simulink model "WaterRocket_uebung"  (Simulink 8.9)
settings: Solver=ode45  StartTime=0.0  StopTime=20  FixedStep=0.000001  RelTol=1e-3  EnableMultiTasking=on
values from neighbouring files (symbols this model uses):
  A = [0 1 0;0 0 1; 0 0 0]    [KalmanBSP.m]    (also in ReadARISData.m = [0 1 0 0 0; 0 0 1 0 0; 0 0 0 0 0;0 0 0 0 0;-0.00649 0 0 0 0]; SEFromData.m = [0 1 0 0 0; SEFromDataWithGPS.m; SEFromDataWithPressure.m = [0 1 0 0 0 0;0 0 1 0 0 0; 0 0 0 0 0 0;0 PressLookUp(1,1) 0 0)
  airdensity = 1.204    [Wasserrakete_uebung.m]
  cw = 0.4    [Wasserrakete_uebung.m]
  F = 0.01^2*pi    (= 0.000314159265359)    [Wasserrakete_uebung.m]
  g = 9.807    [CalcPressure.m]    (also in KalmanBSP.m = 9.81; Wasserrakete_uebung.m = 9.81)
  h0 = 0.3    [Wasserrakete_uebung.m]
  kappa = 1.35    [Wasserrakete_uebung.m]
  ml = 0.113    [Wasserrakete_uebung.m]
  mw0 = v_opt*Vl*rho    (= 0)    [Wasserrakete_uebung.m]
  p0 = 4e5    (= 400000)    [Wasserrakete_uebung.m]
  pa = 0.97e5    (= 97000)    [Wasserrakete_uebung.m]
  rho = 1000    [Wasserrakete_uebung.m]
  V0 = Vl-mw0/rho    (= 0.00158)    [Wasserrakete_uebung.m]
  v0 = 0.0    (= 0)    [Wasserrakete_uebung.m]
  Vl = 1.58e-3    (= 0.00158)    [Wasserrakete_uebung.m]
settings Model: Creator=Benedikt Imbach  LastModifiedBy=Beda Föhn
settings OptimizationCC: InitFltsAndDblsToZero=on
settings DebuggingCC: SaveWithParameterizedLinksMsg=none  SolverPrmCheckMsg=warning
settings HardwareCC: TargetHWDeviceType=32-bit Generic
settings GRTTargetCC: TargetFcnLib=ansi_tfl_tmw.mat  GeneratePreprocessorConditionals=Use local settings

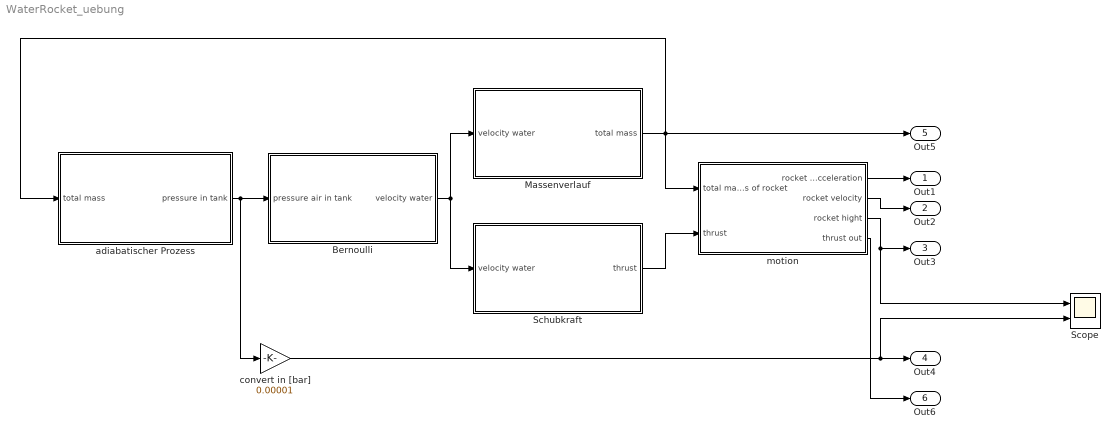
== system WaterRocket_uebung ==
  Bernoulli : Subsystem
  Massenverlauf : Subsystem
  Schubkraft : Subsystem
  Scope : Scope  NumInputPorts=2
  adiabatischer Prozess : Subsystem
  convert in [bar] : Gain  Gain=0.00001
  motion : Subsystem
  Out1 : Outport
  Out2 : Outport  Port=2
  Out3 : Outport  Port=3
  Out4 : Outport  Port=4
  Out5 : Outport  Port=5
  Out6 : Outport  Port=6
  wires:
  adiabatischer Prozess/1(pressure in tank) -> Bernoulli/1(pressure air in tank), convert in [bar]/1
  Bernoulli/1(velocity water) -> Massenverlauf/1(velocity water), Schubkraft/1(velocity water)
  Massenverlauf/1(total mass) -> motion/1(total mass of rocket), adiabatischer Prozess/1(total mass), Out5/1
  Schubkraft/1(thrust) -> motion/2(thrust)
  motion/1(rocket acceleration) -> Out1/1
  motion/2(rocket velocity) -> Out2/1
  motion/3(rocket hight) -> Scope/1, Out3/1
  motion/4(thrust out) -> Out6/1
  convert in [bar]/1 -> Scope/2, Out4/1

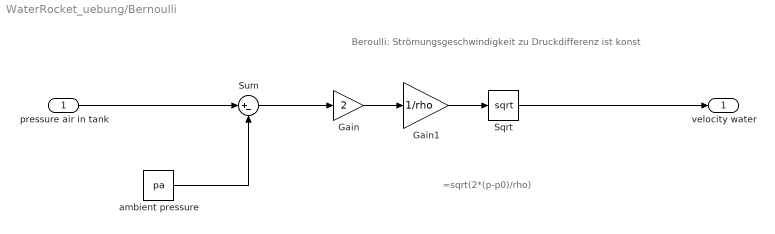
== system WaterRocket_uebung/Bernoulli ==
  note: =sqrt(2*(p-p0)/rho)
  note: Beroulli: Strömungsgeschwindigkeit zu Druckdifferenz ist konst
  pressure air in tank : Inport
  Gain : Gain  Gain=2
  Gain1 : Gain  Gain=1/rho
  Sqrt : Sqrt  SaturateOnIntegerOverflow=on
  Sum : Sum  Inputs=|+-
  ambient pressure : Constant  Value=pa
  velocity water : Outport
  wires:
  pressure air in tank/1 -> Sum/1
  ambient pressure/1 -> Sum/2
  Sum/1 -> Gain/1
  Gain/1 -> Gain1/1
  Gain1/1 -> Sqrt/1
  Sqrt/1 -> velocity water/1

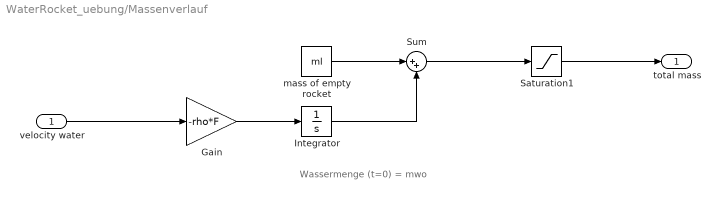
== system WaterRocket_uebung/Massenverlauf ==
  note: Wassermenge (t=0) = mwo
  velocity water : Inport
  Gain : Gain  Gain=-rho*F
  Integrator : Integrator  InitialCondition=mw0
  Saturation1 : Saturate  UpperLimit=ml+mw0  LowerLimit=ml
  Sum : Sum  Inputs=|++
  mass of empty rocket : Constant  Value=ml
  total mass : Outport
  wires:
  velocity water/1 -> Gain/1
  Gain/1 -> Integrator/1
  mass of empty rocket/1 -> Sum/1
  Integrator/1 -> Sum/2
  Sum/1 -> Saturation1/1
  Saturation1/1 -> total mass/1

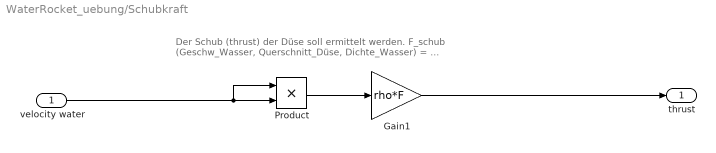
== system WaterRocket_uebung/Schubkraft ==
  note: Der Schub (thrust) der Düse soll ermittelt werden.
      | F_schub (Geschw_Wasser, Querschnitt_Düse, Dichte_Wasser) = ...
  velocity water : Inport
  Gain1 : Gain  Gain=rho*F
  Product : Product
  thrust : Outport
  wires:
  velocity water/1 -> Product/1, Product/2
  Gain1/1 -> thrust/1
  Product/1 -> Gain1/1

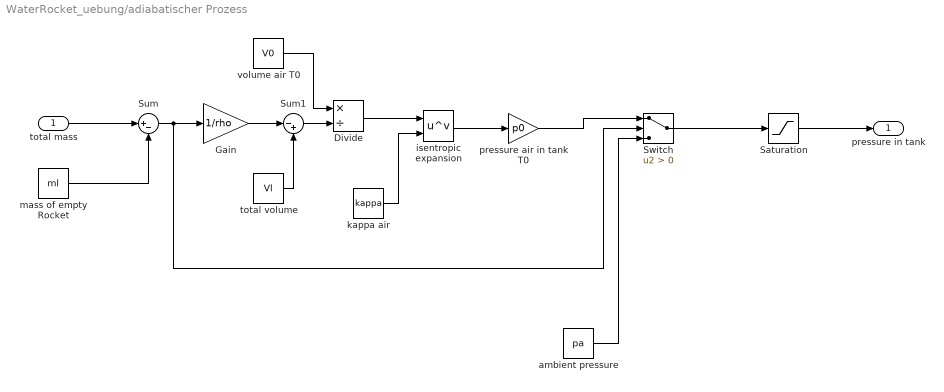
== system WaterRocket_uebung/adiabatischer Prozess ==
  total mass : Inport
  Divide : Product  Inputs=*/
  Gain : Gain  Gain=1/rho
  Saturation : Saturate  UpperLimit=p0  LowerLimit=pa
  Sum : Sum  Inputs=|+-
  Sum1 : Sum  Inputs=|-+
  Switch : Switch  Criteria=u2 > Threshold
  ambient pressure : Constant  Value=pa
  isentropic expansion : Math  Operator=pow  SaturateOnIntegerOverflow=on
  kappa air : Constant  Value=kappa
  mass of empty Rocket : Constant  Value=ml
  pressure air in tank T0 : Gain  Gain=p0
  total volume : Constant  Value=Vl
  volume air T0 : Constant  Value=V0
  pressure in tank : Outport
  wires:
  total mass/1 -> Sum/1
  Sum/1 -> Gain/1, Switch/2
  Gain/1 -> Sum1/1
  Sum1/1 -> Divide/2
  Divide/1 -> isentropic expansion/1
  isentropic expansion/1 -> pressure air in tank T0/1
  mass of empty Rocket/1 -> Sum/2
  total volume/1 -> Sum1/2
  volume air T0/1 -> Divide/1
  kappa air/1 -> isentropic expansion/2
  Saturation/1 -> pressure in tank/1
  pressure air in tank T0/1 -> Switch/1
  Switch/1 -> Saturation/1
  ambient pressure/1 -> Switch/3

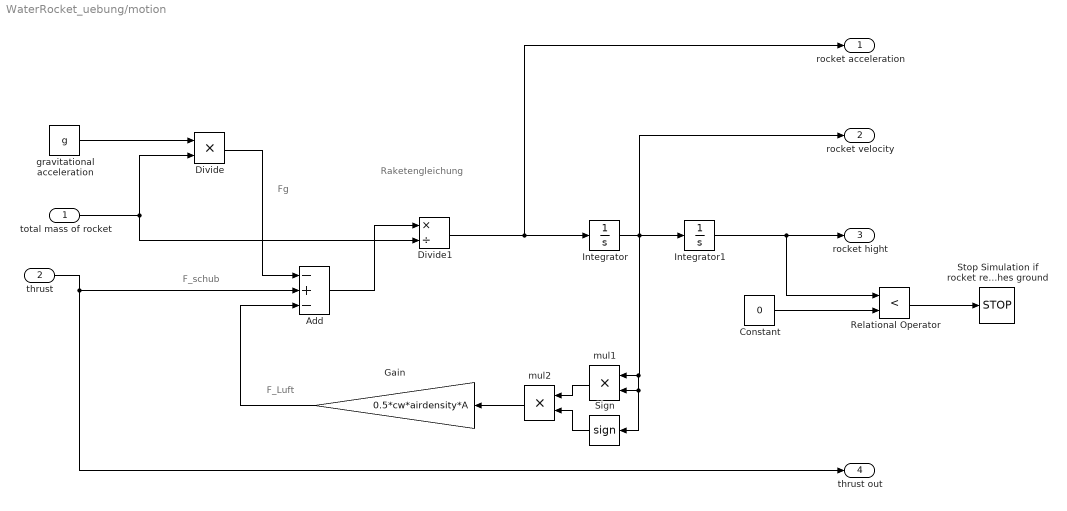
== system WaterRocket_uebung/motion ==
  note: F_Luft
  note: F_schub
  note: Fg
  note: Raketengleichung
  total mass of rocket : Inport
  thrust : Inport  Port=2
  Add : Sum  Inputs=-+-
  Constant : Constant  Value=0
  Divide : Product  Inputs=**
  Divide1 : Product  Inputs=*/
  Gain : Gain  Gain=0.5*cw*airdensity*A
  Integrator : Integrator  InitialCondition=v0
  Integrator1 : Integrator  InitialCondition=h0
  Relational Operator : RelationalOperator  Operator=<  OutDataTypeStr=boolean  RndMeth=Simplest
  Sign : Signum
  Stop Simulation if rocket reaches ground : Stop
  gravitational acceleration : Constant  Value=g
  mul1 : Product  Inputs=**
  mul2 : Product  Inputs=**
  rocket acceleration : Outport
  rocket velocity : Outport  Port=2
  rocket hight : Outport  Port=3
  thrust out : Outport  Port=4
  wires:
  thrust/1 -> thrust out/1, Add/2
  Integrator/1 -> Sign/1, mul1/2, mul1/1, rocket velocity/1, Integrator1/1
  Integrator1/1 -> Relational Operator/1, rocket hight/1
  gravitational acceleration/1 -> Divide/1
  total mass of rocket/1 -> Divide/2, Divide1/2
  Divide/1 -> Add/1
  Gain/1 -> Add/3
  mul1/1 -> mul2/1
  Sign/1 -> mul2/2
  mul2/1 -> Gain/1
  Relational Operator/1 -> Stop Simulation if rocket reaches ground/1
  Constant/1 -> Relational Operator/2
  Add/1 -> Divide1/1
  Divide1/1 -> rocket acceleration/1, Integrator/1
